simulink model "vertical_smm_3d_with_xz_lqr_with_torque_cmds"  (R2015a)
settings: Solver=FixedStepDiscrete  SolverMode=SingleTasking  StartTime=0.0  StopTime=inf  FixedStep=sample_time  RelTol=1e-3
values from neighbouring files (symbols this model uses):
  forward_dx_of_dxstar = [-1.33147741515 -1.28147741462 -1.23147741409 -1.18147741356 -1.13147741303 -1.0814774125 -1.03147741197 -0.981477411445 -0.931477410916 -0.881477410388 -0.831477409975 -0.781477409737 ... (28413 elements, 41x21x33)]    [ref_trajs.mat]
  forward_x_of_dxstar = [0.245075236011 0.237749717983 0.230424199955 0.223098681927 0.215773163898 0.20844764587 0.201122127842 0.193796609813 0.186471091785 0.179145573757 0.171820055745 0.164494537786 ... (28413 elements, 41x21x33)]    [ref_trajs.mat]
  target_dx_range = [-1 -0.95 -0.9 -0.85 -0.8 -0.75 -0.7 -0.65 -0.6 -0.55 -0.5 -0.45 ... (41 elements, 1x41)]    [ref_trajs.mat]
undefined symbols (not defined in the file or in its folder): A_kalman_fourbar_gear, A_kalman_transverse, A_kalman_vertical, A_lpf_accelerometer, A_lpf_dtau, A_lpf_fourbar_angles, A_lpf_imu, A_lpf_lateral_angle, A_lpf_leg_spring, B1_lpf_accelerometer, B1_lpf_dtau, B1_lpf_fourbar_angles, B1_lpf_imu, B1_lpf_lateral_angle, B1_lpf_leg_spring, B2_lpf_accelerometer, B2_lpf_dtau, B2_lpf_fourbar_angles, B2_lpf_imu, B2_lpf_lateral_angle, B2_lpf_leg_spring, B_dx_versus_x0, B_kalman_fourbar_gear, B_kalman_transverse, B_kalman_vertical, backwards_K_sag_of_t, backwards_P_sag_of_t, C_kalman_fourbar_gear, C_kalman_transverse, C_kalman_vertical, com_leg_motor, com_torso, contact_threshold, control_start_time, d_ankle_to_foot, d_vertical_com, desired_com_forward_velocity, desired_com_lateral_velocity, desired_initial_leg_roll_left, desired_initial_leg_roll_right, desired_stance_beta2, desired_standing_torso_pitch, desired_standing_torso_roll, desired_standing_z, desired_torso_pitch, desired_torso_roll, Discrete, enable_bouncing, enable_hopping, fcut_contact, g, HIP_MTR_MAX_CONT_TORQUE, HIP_MTR_MAX_TORQUE, i_leg_motor, i_robot, i_torso, initial_dx_estimate, initial_dy_estimate, initial_dz_estimate, initial_leg_selection ... (+77)
libraries: simulink x18, ctrlSharedLib x7
(part 3 of 5)

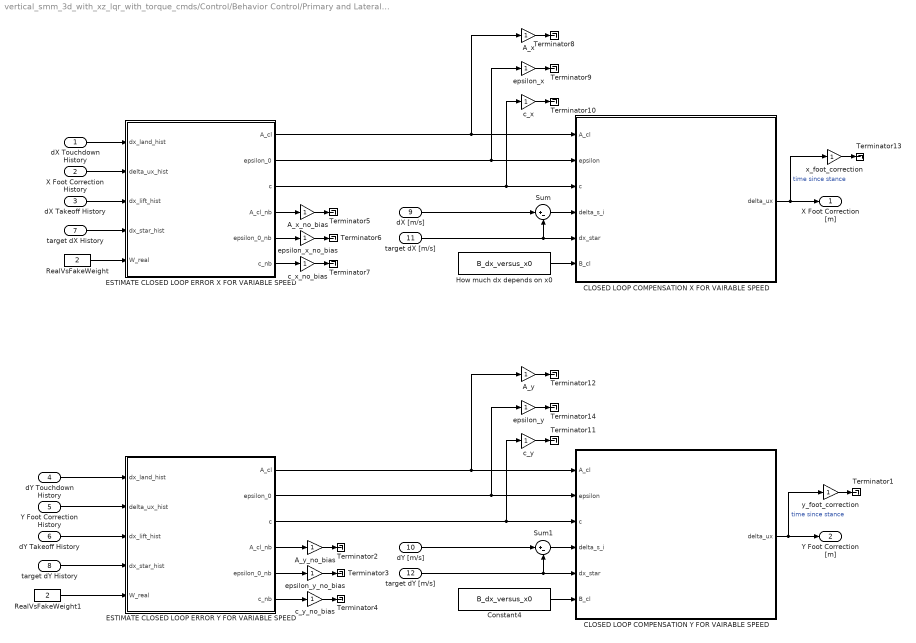
== system vertical_smm_3d_with_xz_lqr_with_torque_cmds/Control/Behavior Control/Primary and Lateral Behavior/Closed Loop Compensation ==
  dX Touchdown History : Inport
  X Foot Correction History : Inport  Port=2
  dX Takeoff History : Inport  Port=3
  dY Touchdown History : Inport  Port=4
  Y Foot Correction History : Inport  Port=5
  dY Takeoff History : Inport  Port=6
  target dX History : Inport  Port=7
  target dY History : Inport  Port=8
  dX [m/s] : Inport  Port=9
  dY [m/s] : Inport  Port=10
  target dX [m/s] : Inport  Port=11
  "target dY [m/s] " : Inport  Port=12
  A_x : Gain
  A_x_no_bias : Gain
  A_y : Gain
  A_y_no_bias : Gain
  CLOSED LOOP COMPENSATION X FOR VAIRABLE SPEED : MATLAB Function  TreatAsAtomicUnit=on
  CLOSED LOOP COMPENSATION Y FOR VAIRABLE SPEED : MATLAB Function  TreatAsAtomicUnit=on
  Constant4 : Constant  Value=B_dx_versus_x0
  ESTIMATE CLOSED LOOP ERROR X FOR VARIABLE SPEED : MATLAB Function  TreatAsAtomicUnit=on
  ESTIMATE CLOSED LOOP ERROR Y FOR VARIABLE SPEED : MATLAB Function  TreatAsAtomicUnit=on
  How much dx depends on x0 : Constant  Value=B_dx_versus_x0
  RealVsFakeWeight : Constant  Value=2
  RealVsFakeWeight1 : Constant  Value=2
  Sum : Sum  Inputs=|+-
  Sum1 : Sum  Inputs=|+-
  Terminator{1..14} (14 alike) : Terminator
  c_x : Gain
  c_x_no_bias : Gain
  c_y : Gain
  c_y_no_bias : Gain
  epsilon_x : Gain
  epsilon_x_no_bias : Gain
  epsilon_y : Gain
  epsilon_y_no_bias : Gain
  x_foot_correction : Gain
  y_foot_correction : Gain
  X Foot Correction [m] : Outport
  Y Foot Correction [m] : Outport  Port=2
  wires:
  RealVsFakeWeight1/1 -> ESTIMATE CLOSED LOOP ERROR Y FOR VARIABLE SPEED/5(W_real)
  Constant4/1 -> CLOSED LOOP COMPENSATION Y FOR VAIRABLE SPEED/6(B_cl)
  "target dY [m/s] "/1 -> Sum1/2, CLOSED LOOP COMPENSATION Y FOR VAIRABLE SPEED/5(dx_star)
  target dY History/1 -> ESTIMATE CLOSED LOOP ERROR Y FOR VARIABLE SPEED/4(dx_star_hist)
  Y Foot Correction History/1 -> ESTIMATE CLOSED LOOP ERROR Y FOR VARIABLE SPEED/2(delta_ux_hist)
  dY Takeoff History/1 -> ESTIMATE CLOSED LOOP ERROR Y FOR VARIABLE SPEED/3(dx_lift_hist)
  dY [m/s]/1 -> Sum1/1
  RealVsFakeWeight/1 -> ESTIMATE CLOSED LOOP ERROR X FOR VARIABLE SPEED/5(W_real)
  How much dx depends on x0/1 -> CLOSED LOOP COMPENSATION X FOR VAIRABLE SPEED/6(B_cl)
  Sum/1 -> CLOSED LOOP COMPENSATION X FOR VAIRABLE SPEED/4(delta_s_i)
  target dX [m/s]/1 -> Sum/2, CLOSED LOOP COMPENSATION X FOR VAIRABLE SPEED/5(dx_star)
  target dX History/1 -> ESTIMATE CLOSED LOOP ERROR X FOR VARIABLE SPEED/4(dx_star_hist)
  X Foot Correction History/1 -> ESTIMATE CLOSED LOOP ERROR X FOR VARIABLE SPEED/2(delta_ux_hist)
  dX Takeoff History/1 -> ESTIMATE CLOSED LOOP ERROR X FOR VARIABLE SPEED/3(dx_lift_hist)
  dX Touchdown History/1 -> ESTIMATE CLOSED LOOP ERROR X FOR VARIABLE SPEED/1(dx_land_hist)
  dX [m/s]/1 -> Sum/1
  dY Touchdown History/1 -> ESTIMATE CLOSED LOOP ERROR Y FOR VARIABLE SPEED/1(dx_land_hist)
  Sum1/1 -> CLOSED LOOP COMPENSATION Y FOR VAIRABLE SPEED/4(delta_s_i)
  CLOSED LOOP COMPENSATION X FOR VAIRABLE SPEED/1(delta_ux) -> x_foot_correction/1, X Foot Correction [m]/1  "time since stance"
  x_foot_correction/1 -> Terminator13/1
  CLOSED LOOP COMPENSATION Y FOR VAIRABLE SPEED/1(delta_ux) -> y_foot_correction/1, Y Foot Correction [m]/1  "time since stance"
  y_foot_correction/1 -> Terminator1/1
  ESTIMATE CLOSED LOOP ERROR X FOR VARIABLE SPEED/6(c_nb) -> c_x_no_bias/1
  ESTIMATE CLOSED LOOP ERROR X FOR VARIABLE SPEED/5(epsilon_0_nb) -> epsilon_x_no_bias/1
  ESTIMATE CLOSED LOOP ERROR X FOR VARIABLE SPEED/4(A_cl_nb) -> A_x_no_bias/1
  A_x_no_bias/1 -> Terminator5/1
  epsilon_x_no_bias/1 -> Terminator6/1
  c_x_no_bias/1 -> Terminator7/1
  A_y_no_bias/1 -> Terminator2/1
  epsilon_y_no_bias/1 -> Terminator3/1
  c_y_no_bias/1 -> Terminator4/1
  ESTIMATE CLOSED LOOP ERROR Y FOR VARIABLE SPEED/4(A_cl_nb) -> A_y_no_bias/1
  ESTIMATE CLOSED LOOP ERROR Y FOR VARIABLE SPEED/5(epsilon_0_nb) -> epsilon_y_no_bias/1
  ESTIMATE CLOSED LOOP ERROR Y FOR VARIABLE SPEED/6(c_nb) -> c_y_no_bias/1
  ESTIMATE CLOSED LOOP ERROR X FOR VARIABLE SPEED/3(c) -> c_x/1, CLOSED LOOP COMPENSATION X FOR VAIRABLE SPEED/3(c)
  ESTIMATE CLOSED LOOP ERROR X FOR VARIABLE SPEED/2(epsilon_0) -> epsilon_x/1, CLOSED LOOP COMPENSATION X FOR VAIRABLE SPEED/2(epsilon)
  ESTIMATE CLOSED LOOP ERROR X FOR VARIABLE SPEED/1(A_cl) -> A_x/1, CLOSED LOOP COMPENSATION X FOR VAIRABLE SPEED/1(A_cl)
  A_x/1 -> Terminator8/1
  epsilon_x/1 -> Terminator9/1
  c_x/1 -> Terminator10/1
  ESTIMATE CLOSED LOOP ERROR Y FOR VARIABLE SPEED/3(c) -> c_y/1, CLOSED LOOP COMPENSATION Y FOR VAIRABLE SPEED/3(c)
  ESTIMATE CLOSED LOOP ERROR Y FOR VARIABLE SPEED/2(epsilon_0) -> epsilon_y/1, CLOSED LOOP COMPENSATION Y FOR VAIRABLE SPEED/2(epsilon)
  ESTIMATE CLOSED LOOP ERROR Y FOR VARIABLE SPEED/1(A_cl) -> A_y/1, CLOSED LOOP COMPENSATION Y FOR VAIRABLE SPEED/1(A_cl)
  A_y/1 -> Terminator12/1
  epsilon_y/1 -> Terminator14/1
  c_y/1 -> Terminator11/1

== system vertical_smm_3d_with_xz_lqr_with_torque_cmds/Control/Behavior Control/Primary and Lateral Behavior/Enabled on Takeoff ==
  In : Inport
  Enable : EnablePort
  Out : Outport
  wires:
  In/1 -> Out/1

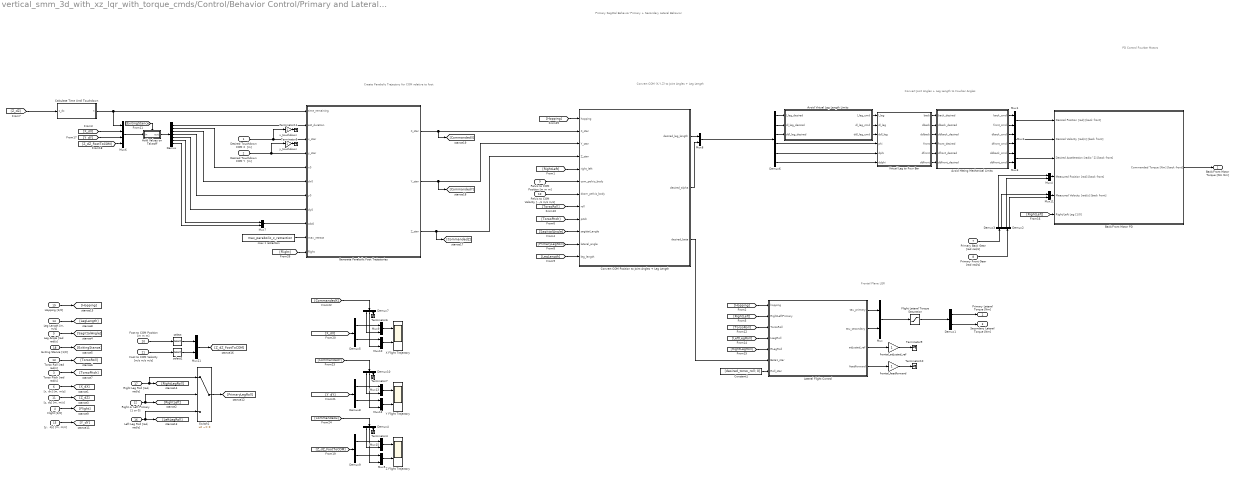
== system vertical_smm_3d_with_xz_lqr_with_torque_cmds/Control/Behavior Control/Primary and Lateral Behavior/Flight ==
  note: Primary Sagittal Behavior
      | Primary + Secondary Lateral Behavior
  note: Create Parabolic
      | Trajectory for COM relative to foot
  note: Convert COM (X,Y,Z) to
      | Joint Angles + Leg Length
  note: Convert Joint Angles + Leg Length
      | to Fourbar Angles
  note: PD Control Fourbar Motors
  note: Frontal Plane LQR
  Desired Touchdown COM X  [m] : Inport
  Desired Touchdown COM Y  [m] : Inport  Port=2
  Torso Pitch [rad rad/s] : Inport  Port=3
  Flight [1/0] : Inport  Port=4
  Leg Angle [rad rad/s] : Inport  Port=5
  "[x, dx] [m, m/s]" : Inport  Port=6
  Primary Back Gear [rad rad/s] : Inport  Port=7
  Primary Front Gear [rad rad/s] : Inport  Port=8
  Pelvis to COM Position [m m m] : Inport  Port=9
  Pelvis to COM Velocity [m/s m/s m/s] : Inport  Port=10
  "[z, dz] [m, m/s]" : Inport  Port=11
  Right or Left Primary [1 or 0] : Inport  Port=12
  Torso Roll [rad rad/s] : Inport  Port=13
  "Leg Length [m, m/s]" : Inport  Port=14
  "[y,  dy] [m, m/s]" : Inport  Port=15
  "Left Leg Roll [rad, rad/s]" : Inport  Port=16
  "Right Leg Roll [rad, rad/s]" : Inport  Port=17
  Exiting Stance [1/0] : Inport  Port=18
  Hopping [1/0] : Inport  Port=19
  Foot to COM Position [m m m] : Inport  Port=20
  Foot to COM Velocity [m/s m/s m/s] : Inport  Port=21
  Avoid Hitting Mechanical Limits : MATLAB Function  TreatAsAtomicUnit=on
  Avoid Virtual Leg Length Limits : MATLAB Function  TreatAsAtomicUnit=on
  Back/Front Motor PD : Subsystem
  Calculate Time Until Touchdown : MATLAB Function  TreatAsAtomicUnit=on
  Constant1 : Constant  Value=[desired_torso_roll; 0]
  "Convert COM Position to Joint Angles + Leg Length " : MATLAB Function  TreatAsAtomicUnit=on
  Demux : Demux  Outputs=7
  Demux{1..3,5,8..9} (6 alike) : Demux  Outputs=2
  Demux10 : Demux  Outputs=3
  Demux4 : Demux  Outputs=3
  Demux6 : Demux  Outputs=6
  Demux7 : Demux  Outputs=3
  Flight Lateral Torque Saturation : Saturate  UpperLimit=HIP_MTR_MAX_CONT_TORQUE  LowerLimit=-HIP_MTR_MAX_CONT_TORQUE
      settings: AttributesFormatString=Top: %<UpperLimit>\nBottom: %<LowerLimit>
  Generate Parabolic Foot Trajectories : MATLAB Function  TreatAsAtomicUnit=on
  Hold Values on Takeoff : Subsystem
  Lateral Flight Control : MATLAB Function  TreatAsAtomicUnit=on
  Mux{,1..5,7..13,15,21} (15 alike) : Mux  Inputs=2
  Mux6 : Mux
  Switch1 : Switch  Criteria=u2 ~= 0
  Terminator{4..7,9..11} (7 alike) : Terminator
  Virtual Leg to Four Bar : MATLAB Function  TreatAsAtomicUnit=on
  X Flight Trajectory : Scope  NumInputPorts=2
      settings: YMin=-1~-0.8  YMax=1~1.4  SaveName=ScopeData3  SampleInput=on
  Y Flight Trajectory : Scope  NumInputPorts=2
      settings: YMin=-1~-0.8  YMax=1~1.4  SaveName=ScopeData4  SampleInput=on
  Z Flight Trajectory : Scope  NumInputPorts=2
      settings: YMin=-1~-0.8  YMax=1~1.4  SaveName=ScopeData7  SampleInput=on
  frontal_adjusted_ref : Gain
  frontal_feedforward : Gain
  max z retraction : Constant  Value=max_parabolic_z_retraction
  select : Selector  InputPortWidth=3  Indices=[3]
  select1 : Selector  InputPortWidth=3  Indices=[3]
  x_touchdown : Gain
  y_touchdown : Gain
  Back/Front Motor Torque [Nm Nm] : Outport
  Primary Lateral Torque [Nm] : Outport  Port=2
  Secondary Lateral Torque [Nm] : Outport  Port=3
  wires:
  Virtual Leg to Four Bar/1(back) -> Avoid Hitting Mechanical Limits/1(back_desired)
  Virtual Leg to Four Bar/2(dback) -> Avoid Hitting Mechanical Limits/2(dback_desired)
  Virtual Leg to Four Bar/3(ddback) -> Avoid Hitting Mechanical Limits/3(ddback_desired)
  Virtual Leg to Four Bar/4(front) -> Avoid Hitting Mechanical Limits/4(front_desired)
  Virtual Leg to Four Bar/5(dfront) -> Avoid Hitting Mechanical Limits/5(dfront_desired)
  Virtual Leg to Four Bar/6(ddfront) -> Avoid Hitting Mechanical Limits/6(ddfront_desired)
  Mux11/1 -> Back/Front Motor PD/5(Measured Velocity [rad/s] [back front])
  Demux2/2 -> Mux11/2
  Mux4/1 -> Back/Front Motor PD/4(Measured Position [rad] [back front])
  Mux1/1 -> Back/Front Motor PD/1(Desired Position [rad] [back front])
  Demux3/2 -> Mux11/1
  Demux3/1 -> Mux4/1
  Avoid Hitting Mechanical Limits/2(front_cmd) -> Mux1/2
  Avoid Hitting Mechanical Limits/1(back_cmd) -> Mux1/1
  Demux2/1 -> Mux4/2
  Avoid Hitting Mechanical Limits/3(dback_cmd) -> Mux2/1
  Avoid Hitting Mechanical Limits/4(dfront_cmd) -> Mux2/2
  Avoid Hitting Mechanical Limits/5(ddback_cmd) -> Mux3/1
  Avoid Hitting Mechanical Limits/6(ddfront_cmd) -> Mux3/2
  Mux2/1 -> Back/Front Motor PD/2(Desired Velocity [rad/s] [back front])
  Mux3/1 -> Back/Front Motor PD/3(Desired Acceleration [rad/s^2] [back front])
  Back/Front Motor PD/1(Commanded Torque [Nm] [back front]) -> Back/Front Motor Torque [Nm Nm]/1
  Primary Back Gear [rad rad/s]/1 -> Demux3/1
  Primary Front Gear [rad rad/s]/1 -> Demux2/1
  [RightLeft] -> Back/Front Motor PD/6(Right/Left Leg [1/0])
  Demux/1 -> Generate Parabolic Foot Trajectories/2(est_duration)
  Mux7/1 -> Generate Parabolic Foot Trajectories/9(zdz0)
  max z retraction/1 -> Generate Parabolic Foot Trajectories/10(max_retract)
  Mux6/1 -> Hold Values on Takeoff/1(in)
  Hold Values on Takeoff/1(out) -> Demux/1
  [X_dX] -> Mux6/2
  Generate Parabolic Foot Trajectories/1(X_star) -> [CommandedX], "Convert COM Position to Joint Angles + Leg Length "/2(X_star)
  Generate Parabolic Foot Trajectories/2(Y_star) -> "Convert COM Position to Joint Angles + Leg Length "/3(Y_star), [CommandedY]
  [RightLeft] -> "Convert COM Position to Joint Angles + Leg Length "/5(right_left)
  "Convert COM Position to Joint Angles + Leg Length "/2(desired_alpha) -> Mux8/2
  "Convert COM Position to Joint Angles + Leg Length "/1(desired_leg_length) -> Mux8/1
  Demux6/6 -> Virtual Leg to Four Bar/6(ddphi)
  Demux6/5 -> Virtual Leg to Four Bar/5(dphi)
  Demux6/4 -> Virtual Leg to Four Bar/4(phi)
  Mux8/1 -> Demux6/1
  Leg Angle [rad rad/s]/1 -> [SagittalAngle]
  [SagittalAngle] -> "Convert COM Position to Joint Angles + Leg Length "/10(sagittal_angle)
  Torso Pitch [rad rad/s]/1 -> [TorsoPitch]
  [TorsoPitch] -> "Convert COM Position to Joint Angles + Leg Length "/9(pitch)
  [PrimaryLegRoll] -> "Convert COM Position to Joint Angles + Leg Length "/11(lateral_angle)
  [LegLength] -> "Convert COM Position to Joint Angles + Leg Length "/12(leg_length)
  [TorsoRoll] -> "Convert COM Position to Joint Angles + Leg Length "/8(roll)
  Pelvis to COM Position [m m m]/1 -> "Convert COM Position to Joint Angles + Leg Length "/6(com_pelvis_body)
  Pelvis to COM Velocity [m/s m/s m/s]/1 -> "Convert COM Position to Joint Angles + Leg Length "/7(dcom_pelvis_body)
  Flight [1/0]/1 -> [Flight]
  [ExitingStance] -> Hold Values on Takeoff/Trigger
  "[x, dx] [m, m/s]"/1 -> [X_dX]
  Torso Roll [rad rad/s]/1 -> [TorsoRoll]
  "Leg Length [m, m/s]"/1 -> [LegLength]
  "[z, dz] [m, m/s]"/1 -> [Z_dZ]
  Desired Touchdown COM X  [m]/1 -> Generate Parabolic Foot Trajectories/3(x_star), x_touchdown/1
  x_touchdown/1 -> Terminator11/1
  y_touchdown/1 -> Terminator5/1
  "[y,  dy] [m, m/s]"/1 -> [Y_dY]
  [Y_dY] -> Mux6/3
  [Z_dZ] -> Calculate Time Until Touchdown/1(z_dz)
  Calculate Time Until Touchdown/1(t) -> Mux6/1, Generate Parabolic Foot Trajectories/1(time_remaining)
  Avoid Virtual Leg Length Limits/1(l_leg_cmd) -> Virtual Leg to Four Bar/1(l_leg)
  Avoid Virtual Leg Length Limits/2(dl_leg_cmd) -> Virtual Leg to Four Bar/2(dl_leg)
  Avoid Virtual Leg Length Limits/3(ddl_leg_cmd) -> Virtual Leg to Four Bar/3(ddl_leg)
  Demux6/1 -> Avoid Virtual Leg Length Limits/1(l_leg_desired)
  Demux6/2 -> Avoid Virtual Leg Length Limits/2(dl_leg_desired)
  Demux6/3 -> Avoid Virtual Leg Length Limits/3(ddl_leg_desired)
  Desired Touchdown COM Y  [m]/1 -> y_touchdown/1, Generate Parabolic Foot Trajectories/4(y_star)
  [RightLeft] -> Lateral Flight Control/2(RightLeftPrimary)
  [TorsoRoll] -> Lateral Flight Control/3(TorsoRoll)
  Constant1/1 -> Lateral Flight Control/7(Roll_star)
  Lateral Flight Control/3(adjusted_ref) -> frontal_adjusted_ref/1
  Lateral Flight Control/4(feedforward) -> frontal_feedforward/1
  Lateral Flight Control/2(tau_secondary) -> Mux/2
  Lateral Flight Control/1(tau_primary) -> Mux/1
  "Left Leg Roll [rad, rad/s]"/1 -> Switch1/3, [LeftLegRoll]
  [LeftLegRoll] -> Lateral Flight Control/4(LLegRoll)
  [RightLegRoll] -> Lateral Flight Control/5(RLegRoll)
  "Right Leg Roll [rad, rad/s]"/1 -> Switch1/1, [RightLegRoll]
  Right or Left Primary [1 or 0]/1 -> Switch1/2, [RightLeft]
  Switch1/1 -> [PrimaryLegRoll]
  Exiting Stance [1/0]/1 -> [ExitingStance]
  Demux1/1 -> Primary Lateral Torque [Nm]/1
  Demux1/2 -> Secondary Lateral Torque [Nm]/1
  "Convert COM Position to Joint Angles + Leg Length "/3(desired_beta) -> Lateral Flight Control/6(Beta1_star)
  Flight Lateral Torque Saturation/1 -> Demux1/1
  frontal_feedforward/1 -> Terminator10/1
  frontal_adjusted_ref/1 -> Terminator9/1
  [Hopping] -> "Convert COM Position to Joint Angles + Leg Length "/1(hopping)
  Mux/1 -> Flight Lateral Torque Saturation/1
  [Hopping] -> Lateral Flight Control/1(hopping)
  Hopping [1/0]/1 -> [Hopping]
  [Flight] -> Generate Parabolic Foot Trajectories/11(flight)
  Demux/2 -> Generate Parabolic Foot Trajectories/5(x0)
  Demux/3 -> Generate Parabolic Foot Trajectories/6(dx0)
  Demux/4 -> Generate Parabolic Foot Trajectories/7(y0)
  Demux/5 -> Generate Parabolic Foot Trajectories/8(dy0)
  Demux/6 -> Mux7/1
  Demux/7 -> Mux7/2
  Foot to COM Position [m m m]/1 -> select/1
  Foot to COM Velocity [m/s m/s m/s]/1 -> select1/1
  select/1 -> Mux21/1
  select1/1 -> Mux21/2
  Mux21/1 -> [Z_dZ_FootToCOM]
  Mux15/1 -> Z Flight Trajectory/1
  Mux5/1 -> Z Flight Trajectory/2
  [Z_dZ_FootToCOM] -> Mux6/4
  [Z_dZ_FootToCOM] -> Demux9/1
  Demux9/1 -> Mux15/1
  Demux9/2 -> Mux5/1
  Demux4/1 -> Mux15/2
  Demux4/2 -> Mux5/2
  Demux4/3 -> Terminator4/1
  Mux9/1 -> X Flight Trajectory/1
  Mux10/1 -> X Flight Trajectory/2
  Demux5/1 -> Mux9/1
  Demux5/2 -> Mux10/1
  Demux7/1 -> Mux9/2
  Demux7/2 -> Mux10/2
  [X_dX] -> Demux5/1
  Demux7/3 -> Terminator6/1
  Mux13/1 -> Y Flight Trajectory/1
  Mux12/1 -> Y Flight Trajectory/2
  Demux8/1 -> Mux13/1
  Demux8/2 -> Mux12/1
  Demux10/1 -> Mux13/2
  Demux10/2 -> Mux12/2
  [Y_dY] -> Demux8/1
  Demux10/3 -> Terminator7/1
  [CommandedX] -> Demux7/1
  [CommandedY] -> Demux10/1
  [CommandedZ] -> Demux4/1
  Generate Parabolic Foot Trajectories/3(Z_star) -> "Convert COM Position to Joint Angles + Leg Length "/4(Z_star), [CommandedZ]

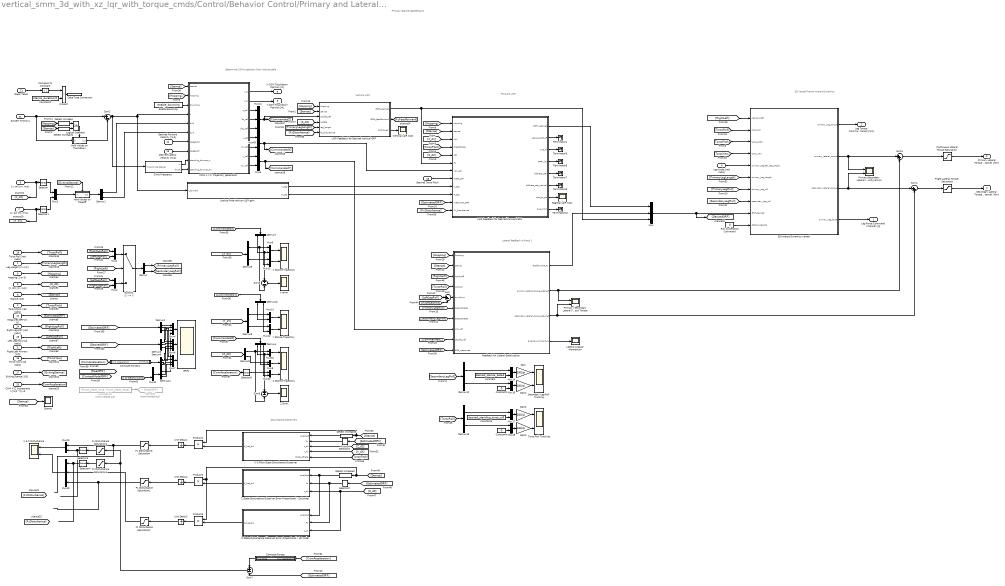
== system vertical_smm_3d_with_xz_lqr_with_torque_cmds/Control/Behavior Control/Primary and Lateral Behavior/Stance ==
  note: Lateral feedback without Y
  note: 3D Yawed Frame Inverse Dynamics
  note: Forward LQR
  note: Vertical LQR
  note: Determine COM trajectory
      | from lookup table
  note: Primary Stance Leg Behavior
  note: Disturbance Observers
  Leg Length [m m/s] : Inport
  Torso Pitch [rad rad/s] : Inport  Port=2
  Stance [1/0] : Inport  Port=3
  Leg Angle [rad rad/s] : Inport  Port=4
  Right/Left Primary [1/0] : Inport  Port=5
  "[x, dx] [m, m/s]" : Inport  Port=6
  "[y, dy] [m, m/s]" : Inport  Port=7
  "[z, dz] [m, m/s]" : Inport  Port=8
  Hopping [1 or 0] : Inport  Port=9
  Measured GRF [N N] : Inport  Port=10
  Steps Taken : Inport  Port=11
  Desired Forward Velocity [m/s] : Inport  Port=12
  Desired Lateral Velocity [m/s] : Inport  Port=13
  Right Leg Roll [rad rad/s] : Inport  Port=14
  Left Leg Roll [rad rad/s] : Inport  Port=15
  Torso Yaw [rad rad/s] : Inport  Port=16
  Exiting Stance [1/0] : Inport  Port=17
  Desired Torso Pitch : Inport  Port=18
  Torso Roll [rad rad/s] : Inport  Port=19
  COM XYZ Acceleration [m/s^2] x3 : Inport  Port=20
  System Time [s] : Inport  Port=21
  3D Inverse Dynamics yawed : MATLAB Function  TreatAsAtomicUnit=on
  COM X,Y,Z  trajectory generation : MATLAB Function  TreatAsAtomicUnit=on
  Chirp Frequency : Subsystem
  Compare To Constant : simulink/Logic and Bit Operations/Compare To Constant  relop=<  const=1  OutDataTypeStr=uint8
  Compute Forces : Subsystem
  Compute Forces1 : Subsystem
  Constant : Constant  Value=desired_stance_beta2
  Constant1 : Constant  Value=0
  Constant2 : Constant  Value=stance_duration/2
  Constant3 : Constant  Value=desired_standing_torso_roll
  Constant4 : Constant  Value=0
  Continuous Lateral Torque Saturation : Saturate  UpperLimit=max_primary_lateral_stance_torque  LowerLimit=-max_primary_lateral_stance_torque
      settings: AttributesFormatString=Top: %<UpperLimit>\nBottom: %<LowerLimit>
  Data Type Conversion : DataTypeConversion  OutDataTypeStr=double
  Demux{,1,5,7..10,12..13} (9 alike) : Demux  Outputs=2
  Demux{2..4,6,11} (5 alike) : Demux  Outputs=3
  Detect Increase{,1..3} (4 alike) : simulink/Logic and Bit Operations/Detect Increase  vinit=0.0  InputProcessing=Inherited  OutDataTypeStr=boolean
  Enable Bouncing : Constant  Value=enable_bouncing  SampleTime=sample_time
  Feedback for Lateral Stabilization : MATLAB Function  TreatAsAtomicUnit=on
  Flight Lateral Torque Saturation : Saturate  UpperLimit=HIP_MTR_MAX_CONT_TORQUE  LowerLimit=-HIP_MTR_MAX_CONT_TORQUE
      settings: AttributesFormatString=Top: %<UpperLimit>\nBottom: %<LowerLimit>
  Fx Disturbance Saturation : Saturate  UpperLimit=100  LowerLimit=-100
      settings: AttributesFormatString=Top: %<UpperLimit>\nBottom: %<LowerLimit>
  Fx Disturbance Saturation1 : Saturate  UpperLimit=100  LowerLimit=-100
      settings: AttributesFormatString=Top: %<UpperLimit>\nBottom: %<LowerLimit>
  Fz Disturbance Saturation1 : Saturate  UpperLimit=100  LowerLimit=-100
      settings: AttributesFormatString=Top: %<UpperLimit>\nBottom: %<LowerLimit>
  Fz Disturbance Saturation2 : Saturate  UpperLimit=100  LowerLimit=-100
      settings: AttributesFormatString=Top: %<UpperLimit>\nBottom: %<LowerLimit>
  Fz Disturbance Saturation4 : Saturate  UpperLimit=100  LowerLimit=-100
      settings: AttributesFormatString=Top: %<UpperLimit>\nBottom: %<LowerLimit>
  GRFs : Scope  NumInputPorts=3
      settings: TimeRange=37.999  YMin=-1250~-2000~-1250  YMax=1500~3750~1750  SampleInput=on
  Gain{,1..3} (4 alike) : Gain  Gain=180/pi
  Hold Values on Takeoff : Subsystem
  Hold Values on Touchdown : Subsystem
  LQR Feedback for Desired Forward GRF : MATLAB Function  TreatAsAtomicUnit=on
  LQR Feedback for Desired Vertical GRF : MATLAB Function  TreatAsAtomicUnit=on
  Lateral Angular Momentum : Scope
      settings: YMin=-3.5  YMax=4  SaveName=ScopeData20  SampleInput=on
  Logical Operator : Logic  Operator=OR  AllPortsSameDT=off  OutDataTypeStr=boolean
  Lookup finite horizon LQR gain : MATLAB Function  TreatAsAtomicUnit=on
  Mux{,11,19,21} (4 alike) : Mux  Inputs=3
  Mux{1..3,5,8..10,12..18,20,22,49} (17 alike) : Mux  Inputs=2
  Mux4 : Mux
  Mux6 : Mux
  Mux7 : Mux
  Primary / Secondary Lateral Feedback Torque : Scope  NumInputPorts=2
      settings: YMin=-3.5~-5  YMax=4~5  SaveName=ScopeData9  SampleInput=on
  Primary/Secondary Lateral Inverse Dynamics : Scope  NumInputPorts=2
      settings: YMin=40~-5  YMax=150~5  SaveName=ScopeData34  SampleInput=on
  Product{,1..3} (4 alike) : Product
  Roll Accleration Command : Constant  Value=0
  Sagittal LQR Cost : Scope
      settings: YMin=22.5  YMax=62.5  SaveName=ScopeData10  SampleInput=on
  Secondary Leg Roll Tracking : Scope  NumInputPorts=2
      settings: YMin=-3.5~-5  YMax=4~5  SaveName=ScopeData12  SampleInput=on
  Selector : Selector  InputPortWidth=2  Indices=[2]
  Selector1 : Selector  InputPortWidth=2  Indices=[2]
  Selector2 : Selector  InputPortWidth=3  Indices=[3]
  Selector3 : Selector  InputPortWidth=3  Indices=[1]
  Selector4 : Selector  InputPortWidth=3  Indices=[3]
  Selector5 : Selector  InputPortWidth=3  Indices=[1]
  Selector6 : Selector  InputPortWidth=3  Indices=[3]
  Stance : Scope
      settings: YMin=-0.05  YMax=0.11  SaveName=stance_time_history  SampleInput=on
  Sum : Sum  Inputs=|+-
  Sum2 : Sum  Inputs=|+-
  Sum3 : Sum  Inputs=|++
  Sum4 : Sum  Inputs=|++
  Sum5 : Sum  Inputs=+-
  Sum6 : Sum  Inputs=+-
  Sum7 : Sum  Inputs=+-
  Switch1 : Switch  Criteria=u2 ~= 0
  Terminator{4..8,10} (6 alike) : Terminator
  Torso Roll Tracking : Scope  NumInputPorts=2
      settings: YMin=-3.5~-5  YMax=4~5  SaveName=ScopeData15  SampleInput=on
  Unit Delay1 : UnitDelay  SampleTime=sample_time
  Unit Delay2 : UnitDelay  SampleTime=sample_time
  Unit Delay3 : UnitDelay  SampleTime=sample_time
  Vertical LQR Cost : Scope
      settings: YMin=11  YMax=16  SaveName=ScopeData18  SampleInput=on
  X & Pitch State Disturbance Observer : MATLAB Function  TreatAsAtomicUnit=on
  X & Z Disturbance : Scope  NumInputPorts=2
      settings: YMin=-125~-800  YMax=175~700  SaveName=ScopeData16  SampleInput=on
  X Stance Trajectory : Scope  NumInputPorts=2
      settings: YMin=0~-0.02  YMax=0.005~0.03  SaveName=ScopeData8  SampleInput=on
  X error : Scope
      settings: YMin=-0.05  YMax=0.11  SaveName=ScopeData24  SampleInput=on
  Y Stance Trajectory : Scope  NumInputPorts=2
      settings: YMin=0.005~-0.5  YMax=0.1~0.3  SaveName=ScopeData5  SampleInput=on
  Z Error : Scope
      settings: YMin=-0.007  YMax=0.0005  SaveName=ScopeData23  SampleInput=on
  Z Stance Trajectory : Scope  NumInputPorts=3
      settings: YMin=0.85~-0.4~-3  YMax=0.98~0.6~11  SaveName=z_stance_trajectory  SampleInput=on
  Z State Disturbance Observer Error-Proportional - 1st order : MATLAB Function  TreatAsAtomicUnit=on
  Z State Disturbance Observer Error-Proportional - 2nd order : MATLAB Function  TreatAsAtomicUnit=on
  recorded q1 : FromWorkspace  Commented=on  VariableName=[force_plate_time, force_plate_data]  OutDataTypeStr=double  OutputAfterFinalValue=Holding final value
  stance20 : Goto  Commented=on  GotoTag=RealGRF
  Leg Force Command (stance) [N] : Outport
  Leg Torque Command (stance) [Nm] : Outport  Port=2
  Primary Lateral Torque Command (stance) [Nm] : Outport  Port=3
  Secondary Lateral Torque Command (stance) [Nm] : Outport  Port=4
  X COM Touchdown Position [m] : Outport  Port=5
  Y COM Touchdown Position [m] : Outport  Port=6
  wires:
  Fz Disturbance Saturation4/1 -> Selector4/1
  Fz Disturbance Saturation1/1 -> Mux19/3
  Fx Disturbance Saturation1/1 -> Selector5/1
  Chirp Frequency/2(dw/dt) -> COM X,Y,Z  trajectory generation/10(standing_bounce_dw)
  [Stance] -> Stance/1
  Chirp Frequency/1(w) -> COM X,Y,Z  trajectory generation/9(standing_bounce_w)
  Selector2/1 -> Z State Disturbance Observer Error-Proportional - 1st order/2(Fz), Z State Disturbance Observer Error-Proportional - 2nd order/2(Fz)
  Sum7/1 -> Fx Disturbance Saturation1/1, Fz Disturbance Saturation4/1
  Unit Delay3/1 -> Fz Disturbance Saturation2/1
  Selector5/1 -> Mux20/2
  Mux20/1 -> X & Z Disturbance/1
  [ComAcceleration] -> Compute Forces/1(XYZ Acceleration)
  Compute Forces/1(XYZ Force) -> Sum7/1
  [FxDisturbance] -> LQR Feedback for Desired Forward GRF/12(Fx_disturbance)
  Sum6/1 -> X error/1
  Demux7/1 -> Mux9/2, Sum6/1
  Demux5/1 -> Mux9/1, Sum6/2
  Unit Delay2/1 -> Fz Disturbance Saturation1/1
  Unit Delay1/1 -> Fx Disturbance Saturation/1
  Selector3/1 -> X & Pitch State Disturbance Observer/2(Fx)
  Fx Disturbance Saturation/1 -> Mux20/1
  Enable Bouncing/1 -> COM X,Y,Z  trajectory generation/3(bouncing)
  [RightLeft] -> Feedback for Lateral Stabilization/3(right_left)
  Constant4/1 -> Mux18/2
  Mux18/1 -> Gain3/1
  Demux13/2 -> Mux18/1
  Constant3/1 -> Mux17/2
  Demux13/1 -> Mux17/1
  Mux17/1 -> Gain2/1
  Gain3/1 -> Torso Roll Tracking/2
  Gain2/1 -> Torso Roll Tracking/1
  [TorsoRoll] -> Demux13/1
  Constant1/1 -> Mux16/2
  Demux12/2 -> Mux16/1
  Mux16/1 -> Gain1/1
  Gain1/1 -> Secondary Leg Roll Tracking/2
  Gain/1 -> Secondary Leg Roll Tracking/1
  Constant/1 -> Mux14/2
  Demux12/1 -> Mux14/1
  Mux14/1 -> Gain/1
  [SecondaryLegRoll] -> Demux12/1
  Feedback for Lateral Stabilization/3(secondary_lateral_torque_desired) -> Sum4/2, Primary / Secondary Lateral Feedback Torque/2
  Sum4/1 -> Flight Lateral Torque Saturation/1
  3D Inverse Dynamics yawed/2(primary_lateral_torque) -> Sum3/1, Primary/Secondary Lateral Inverse Dynamics/1
  3D Inverse Dynamics yawed/3(secondary_lateral_torque) -> Sum4/1, Primary/Secondary Lateral Inverse Dynamics/2
  Sum/1 -> Feedback for Lateral Stabilization/5(symdsym)
  [SecondaryLegRoll] -> Feedback for Lateral Stabilization/7(beta2dbeta2)
  [PrimaryLegRoll] -> Feedback for Lateral Stabilization/6(beta1dbeta1)
  [RightLegRoll] -> Sum/2
  [LeftLegRoll] -> Sum/1
  Feedback for Lateral Stabilization/2(primary_lateral_torque_desired) -> Sum3/2, Primary / Secondary Lateral Feedback Torque/1
  Sum3/1 -> Continuous Lateral Torque Saturation/1
  Roll Accleration Command/1 -> 3D Inverse Dynamics yawed/10(ddRoll_desired)
  Feedback for Lateral Stabilization/1(feedforward_Fy) -> Mux/2
  Continuous Lateral Torque Saturation/1 -> Primary Lateral Torque Command (stance) [Nm]/1
  Demux11/3 -> Mux7/4
  Demux11/2 -> Mux6/4
  Demux11/1 -> Mux4/4
  Mux/1 -> [DesiredGRF], 3D Inverse Dynamics yawed/9(GRF_desired)
  LQR Feedback for Desired Forward GRF/1(GRFx_desired) -> Mux/1
  Left Leg Roll [rad rad/s]/1 -> [LeftLegRoll]
  Right/Left Primary [1/0]/1 -> [RightLeft]
  [CommandedY] -> Demux10/1
  [CommandedX] -> Demux7/1
  [Y_dY] -> Demux8/1
  Demux10/2 -> Mux12/2
  Demux10/1 -> Mux13/2
  Demux8/2 -> Mux12/1
  Demux8/1 -> Mux13/1
  Mux12/1 -> Y Stance Trajectory/2
  Mux13/1 -> Y Stance Trajectory/1
  [X_dX] -> Demux5/1
  Demux7/2 -> Mux10/2
  Demux5/2 -> Mux10/1
  Mux10/1 -> X Stance Trajectory/2
  Mux9/1 -> X Stance Trajectory/1
  Demux3/3 -> Mux7/2
  Demux3/2 -> Mux6/2
  Demux3/1 -> Mux4/2
  Demux2/3 -> Mux7/1
  Demux2/2 -> Mux6/1
  Mux7/1 -> GRFs/3
  Mux6/1 -> GRFs/2
  Demux2/1 -> Mux4/1
  Mux4/1 -> GRFs/1
  [DesiredGRF] -> Demux3/1
  [EstimatedGRF] -> Demux2/1
  Torso Roll [rad rad/s]/1 -> [TorsoRoll]
  [PrimaryLegLength] -> LQR Feedback for Desired Vertical GRF/5(leg_length)
  Leg Length [m m/s]/1 -> [PrimaryLegLength]
  System Time [s]/1 -> Sum2/1, Hold Values on Touchdown/1(in)
  [EstimatedGRF] -> Feedback for Lateral Stabilization/10(GRF_measured)
  [Hopping] -> Feedback for Lateral Stabilization/1(hopping)
  3D Inverse Dynamics yawed/4(primary_leg_force) -> Leg Force Command (stance) [N]/1
  [ExitingStance] -> Hold Values on Takeoff/Trigger
  Exiting Stance [1/0]/1 -> [ExitingStance]
  Torso Yaw [rad rad/s]/1 -> [TorsoYaw]
  Desired Lateral Velocity [m/s]/1 -> COM X,Y,Z  trajectory generation/8(target_DY)
  Selector1/1 -> Mux3/2
  Hold Values on Takeoff/1(out) -> Demux1/1
  Mux3/1 -> Hold Values on Takeoff/1(in)
  "[y, dy] [m, m/s]"/1 -> Selector1/1, [Y_dY]
  [RightLeft] -> Switch1/2
  [RightLegRoll] -> Mux2/2
  [LeftLegRoll] -> Mux2/1
  [LeftLegRoll] -> Mux1/2
  [RightLegRoll] -> Mux1/1
  Right Leg Roll [rad rad/s]/1 -> [RightLegRoll]
  Mux2/1 -> Switch1/3
  Mux1/1 -> Switch1/1
  Demux/1 -> [PrimaryLegRoll]
  Demux/2 -> [SecondaryLegRoll]
  Switch1/1 -> Demux/1
  [PrimaryLegRoll] -> 3D Inverse Dynamics yawed/7(primary_leg_roll)
  [SecondaryLegRoll] -> 3D Inverse Dynamics yawed/8(secondary_leg_roll)
  Leg Angle [rad rad/s]/1 -> 3D Inverse Dynamics yawed/5(primary_sagittal_leg_angle)
  [PrimaryLegLength] -> 3D Inverse Dynamics yawed/6(primary_leg_length)
  [TorsoYaw] -> 3D Inverse Dynamics yawed/4(torso_yaw)
  [TorsoRoll] -> 3D Inverse Dynamics yawed/2(torso_roll)
  [TorsoPitch] -> 3D Inverse Dynamics yawed/3(torso_pitch)
  Mux5/1 -> [CommandedY], Feedback for Lateral Stabilization/8(ydy_ref)
  COM X,Y,Z  trajectory generation/2(y_0) -> Y COM Touchdown Position [m]/1
  [CommandedZ] -> Feedback for Lateral Stabilization/9(zdzddz_ref)
  [TorsoRoll] -> Feedback for Lateral Stabilization/4(rolldroll)
  [Stance] -> Feedback for Lateral Stabilization/2(stance)
  [Hopping] -> LQR Feedback for Desired Vertical GRF/1(hopping)
  Selector/1 -> Mux3/1
  Demux1/1 -> COM X,Y,Z  trajectory generation/5(dx0)
  [Stance] -> Detect Increase1/1
  [Hopping] -> Detect Increase/1
  Compare To Constant/1 -> Product/1
  Detect Increase1/1 -> Logical Operator/2
  Detect Increase/1 -> Logical Operator/1
  Constant2/1 -> Product/2
  Product/1 -> Data Type Conversion/1
  Steps Taken/1 -> Compare To Constant/1
  [EstimatedGRF] -> LQR Feedback for Desired Forward GRF/11(measured_GRF)
  Measured GRF [N N]/1 -> [EstimatedGRF]
  [Hopping] -> LQR Feedback for Desired Forward GRF/1(hopping)
  [Hopping] -> COM X,Y,Z  trajectory generation/2(hopping)
  Hopping [1 or 0]/1 -> [Hopping]
  [RightLeft] -> 3D Inverse Dynamics yawed/1(right_or_left)
  Torso Pitch [rad rad/s]/1 -> [TorsoPitch]
  LQR Feedback for Desired Forward GRF/8(ang_mom) -> Terminator10/1
  LQR Feedback for Desired Forward GRF/7(cost_to_go) -> Sagittal LQR Cost/1
  LQR Feedback for Desired Forward GRF/6(ddtheta_star_neutral) -> Terminator8/1
  LQR Feedback for Desired Forward GRF/5(ddtheta_star) -> Terminator7/1
  LQR Feedback for Desired Forward GRF/3(true_ff) -> Terminator5/1
  LQR Feedback for Desired Forward GRF/2(netural_pitch_ff) -> Terminator4/1
  LQR Feedback for Desired Vertical GRF/3(cost_to_go) -> Vertical LQR Cost/1
  Demux1/2 -> COM X,Y,Z  trajectory generation/6(dy0)
  "[x, dx] [m, m/s]"/1 -> Selector/1, [X_dX]
  Logical Operator/1 -> Hold Values on Touchdown/Trigger
  [Stance] -> LQR Feedback for Desired Vertical GRF/2(stance)
  Stance [1/0]/1 -> [Stance]
  Hold Values on Touchdown/1(out) -> Sum2/2
  LQR Feedback for Desired Vertical GRF/1(GRFz_desired) -> Mux/3, LQR Feedback for Desired Forward GRF/6(Fz)
  Sum2/1 -> COM X,Y,Z  trajectory generation/4(t), Lookup finite horizon LQR gain/1(t_forward), Chirp Frequency/1(Time Since Stance)
  Desired Forward Velocity [m/s]/1 -> COM X,Y,Z  trajectory generation/7(target_DX)
  [Z_dZ] -> LQR Feedback for Desired Forward GRF/5(zdz)
  Lookup finite horizon LQR gain/1(K_sag) -> LQR Feedback for Desired Forward GRF/9(K_sag)
  Desired Torso Pitch/1 -> LQR Feedback for Desired Forward GRF/8(theta_star)
  Mux49/1 -> LQR Feedback for Desired Forward GRF/7(xdx_ref), [CommandedX]
  [TorsoPitch] -> LQR Feedback for Desired Forward GRF/4(thetadtheta)
  [X_dX] -> LQR Feedback for Desired Forward GRF/3(xdx)
  Mux11/1 -> LQR Feedback for Desired Vertical GRF/3(zdzddz_ref), [CommandedZ]
  COM X,Y,Z  trajectory generation/5(ddz_ref) -> Mux11/3
  COM X,Y,Z  trajectory generation/4(dz_ref) -> Mux11/2
  COM X,Y,Z  trajectory generation/1(x_0) -> X COM Touchdown Position [m]/1
  COM X,Y,Z  trajectory generation/9(dy_ref) -> Mux5/2
  COM X,Y,Z  trajectory generation/8(y_ref) -> Mux5/1
  COM X,Y,Z  trajectory generation/7(dx_ref) -> Mux49/2
  COM X,Y,Z  trajectory generation/6(x_ref) -> Mux49/1
  [Stance] -> LQR Feedback for Desired Forward GRF/2(stance)
  COM X,Y,Z  trajectory generation/3(z_ref) -> Mux11/1
  [Z_dZ] -> LQR Feedback for Desired Vertical GRF/4(z_state)
  3D Inverse Dynamics yawed/1(primary_leg_torque) -> Leg Torque Command (stance) [Nm]/1
  Lookup finite horizon LQR gain/2(P_sag) -> LQR Feedback for Desired Forward GRF/10(P_sag)
  [Stance] -> COM X,Y,Z  trajectory generation/1(stance)
  LQR Feedback for Desired Forward GRF/4(GRFx_lqr) -> Terminator6/1
  Feedback for Lateral Stabilization/4(angular_momentum) -> Lateral Angular Momentum/1
  Demux6/1 -> Mux4/3
  Demux6/2 -> Mux6/3
  Demux6/3 -> Mux7/3
  Flight Lateral Torque Saturation/1 -> Secondary Lateral Torque Command (stance) [Nm]/1
  "[z, dz] [m, m/s]"/1 -> [Z_dZ]
  [Z_dZ] -> X & Pitch State Disturbance Observer/3(z_dz)
  [TorsoPitch] -> X & Pitch State Disturbance Observer/5(theta_dtheta)
  [X_dX] -> X & Pitch State Disturbance Observer/4(x_dx)
  [EstimatedGRF] -> Selector3/1
  Detect Increase3/1 -> X & Pitch State Disturbance Observer/1(enabled)
  Detect Increase2/1 -> Z State Disturbance Observer Error-Proportional - 1st order/1(enabled), Z State Disturbance Observer Error-Proportional - 2nd order/1(enabled)
  [EstimatedGRF] -> Selector2/1
  [Z_dZ] -> Z State Disturbance Observer Error-Proportional - 1st order/3(z_dz), Z State Disturbance Observer Error-Proportional - 2nd order/3(z_dz)
  Product1/1 -> Unit Delay1/1
  Product2/1 -> Unit Delay2/1
  X & Pitch State Disturbance Observer/1(d_hat_tp1) -> Product1/2
  [Stance] -> Product1/1, Detect Increase3/1
  Z State Disturbance Observer Error-Proportional - 2nd order/1(d_hat_tp1) -> Product2/2
  Product3/1 -> Unit Delay3/1
  Z State Disturbance Observer Error-Proportional - 1st order/1(d_hat_tp1) -> Product3/2
  [Stance] -> Product3/1, Product2/1, Detect Increase2/1
  Mux19/1 -> X & Z Disturbance/2
  Fz Disturbance Saturation2/1 -> Mux19/2
  [EstimatedGRF] -> Sum7/2
  Selector4/1 -> Mux19/1
  recorded q1/1 -> stance20/1
  COM XYZ Acceleration [m/s^2] x3/1 -> [ComAcceleration]
  [ComAcceleration] -> Compute Forces1/1(XYZ Acceleration)
  Compute Forces1/1(XYZ Force) -> Demux6/1
  [FzDisturbance] -> LQR Feedback for Desired Vertical GRF/6(Fz_disturbance)
  LQR Feedback for Desired Vertical GRF/2(GRFz_feedforward) -> [FzFeedforward]
  Mux21/1 -> Demux11/1
  [FzFeedforward] -> Mux21/3
  Mux15/1 -> Z Stance Trajectory/1
  Mux8/1 -> Z Stance Trajectory/2
  [Z_dZ] -> Demux9/1
  Demux9/1 -> Mux15/1, Sum5/2
  Demux9/2 -> Mux8/1
  Demux4/1 -> Mux15/2, Sum5/1
  Demux4/2 -> Mux8/2
  Demux4/3 -> Mux22/2
  [CommandedZ] -> Demux4/1
  Sum5/1 -> Z Error/1
  Mux22/1 -> Z Stance Trajectory/3
  [ComAcceleration] -> Selector6/1
  Selector6/1 -> Mux22/1

== system vertical_smm_3d_with_xz_lqr_with_torque_cmds/Control/Behavior Control/Secondary Leg Behavior/Back//Front Motor PD ==
  Desired Position [rad] [back front] : Inport
  Desired Velocity [rad/s] [back front] : Inport  Port=2
  Desired Acceleration [rad/s^2] [back front] : Inport  Port=3
  Measured Position [rad] [back front] : Inport  Port=4
  Measured Velocity [rad/s] [back front] : Inport  Port=5
  Right/Left Leg [1/0] : Inport  Port=6
  Divide : Product  Inputs=*/
  Friction Compensation : Subsystem
  Load Torque in Flight : Constant  Value=30
  Motor Efficiency : MATLAB Function  TreatAsAtomicUnit=on
  Product : Product
  RPM in Flight : Constant  Value=0
  Sum1 : Sum  Inputs=|++
  Sum2 : Sum  Inputs=|++
  Sum7 : Sum  Inputs=|+-
  Sum8 : Sum  Inputs=|+-
  Sum9 : Sum
  kd : Gain  Gain=kd_motor
  kp : Gain  Gain=kp_motor
  reflected inertia : Constant  Value=j_motor
  Commanded Torque [Nm] [back front] : Outport
  wires:
  kp/1 -> Sum9/1
  Sum7/1 -> kp/1
  Measured Position [rad] [back front]/1 -> Sum7/2
  Sum9/1 -> Sum1/1
  Sum8/1 -> kd/1
  Desired Position [rad] [back front]/1 -> Sum7/1
  kd/1 -> Sum9/2
  Measured Velocity [rad/s] [back front]/1 -> Sum8/2
  Desired Acceleration [rad/s^2] [back front]/1 -> Product/1
  Product/1 -> Sum1/2
  Right/Left Leg [1/0]/1 -> Friction Compensation/1(Right/Left [1/0])
  Sum2/1 -> Commanded Torque [Nm] [back front]/1
  Desired Velocity [rad/s] [back front]/1 -> Friction Compensation/2(Commanded Velocity [rad/s] [back front]), Sum8/1
  reflected inertia/1 -> Product/2
  RPM in Flight/1 -> Motor Efficiency/1(rpm)
  Motor Efficiency/1(mu) -> Divide/2
  Divide/1 -> Sum2/1
  Sum1/1 -> Divide/1
  Load Torque in Flight/1 -> Motor Efficiency/2(load_torque)

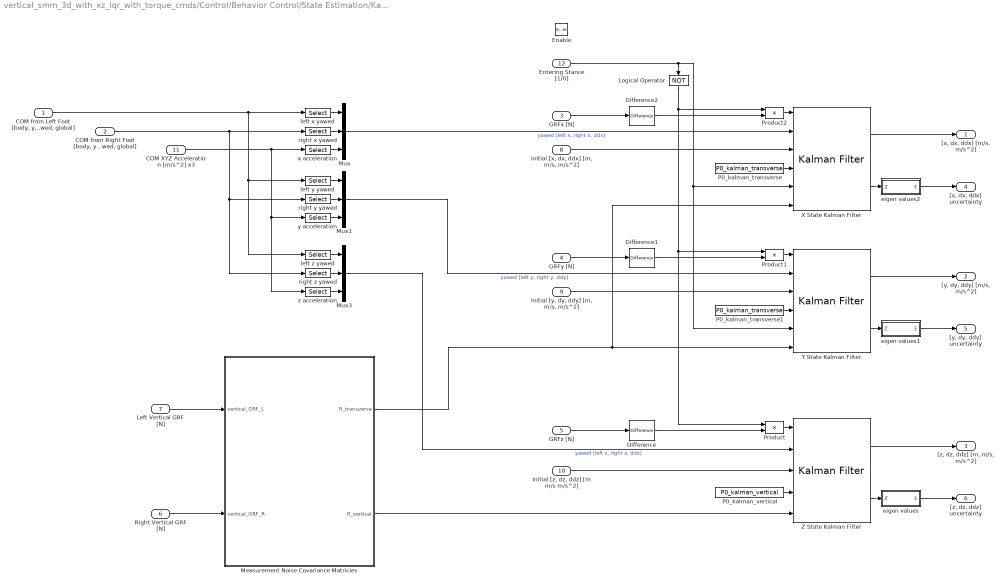
== system vertical_smm_3d_with_xz_lqr_with_torque_cmds/Control/Behavior Control/State Estimation/Kalman Filtering ==
  "COM from Left Foot [body, yawed, global]" : Inport  SampleTime=sample_time
  "COM from Right Foot [body, yawed, global]" : Inport  Port=2  SampleTime=sample_time
  GRFx [N] : Inport  Port=3  SampleTime=sample_time
  GRFy [N] : Inport  Port=4  SampleTime=sample_time
  GRFz [N] : Inport  Port=5  SampleTime=sample_time
  Right Vertical GRF [N] : Inport  Port=6  SampleTime=sample_time
  Left Vertical GRF [N] : Inport  Port=7  SampleTime=sample_time
  "Initial [x, dx, ddx] [m, m/s, m/s^2]" : Inport  Port=8  PortDimensions=3  SampleTime=sample_time
  "Initial [y, dy, ddy] [m, m/s, m/s^2]" : Inport  Port=9  PortDimensions=3  SampleTime=sample_time
  "Initial [z, dz, ddz] [m m/s m/s^2]" : Inport  Port=10  PortDimensions=3  SampleTime=sample_time
  COM XYZ Acceleration [m/s^2] x3 : Inport  Port=11  SampleTime=sample_time
  Entering Stance [1/0] : Inport  Port=12  PortDimensions=1  SampleTime=sample_time
  Enable : EnablePort  StatesWhenEnabling=reset
  Difference : simulink/Discrete/Difference  ICPrevInput=0.0  InputProcessing=Inherited  OutMin=[]  OutMax=[]  OutDataType=fixdt(1, 16)  OutScaling=2^-10  DoSatur=off
  Difference1 : simulink/Discrete/Difference  ICPrevInput=0.0  InputProcessing=Inherited  OutMin=[]  OutMax=[]  OutDataType=fixdt(1, 16)  OutScaling=2^-10  DoSatur=off
  Difference2 : simulink/Discrete/Difference  ICPrevInput=0.0  InputProcessing=Inherited  OutMin=[]  OutMax=[]  OutDataType=fixdt(1, 16)  OutScaling=2^-10  DoSatur=off
  Logical Operator : Logic  Operator=NOT  AllPortsSameDT=off  OutDataTypeStr=boolean
  Measurement Noise Covariance Matricies : MATLAB Function  TreatAsAtomicUnit=on
  Mux : Mux  Inputs=3
  Mux1 : Mux  Inputs=3
  Mux3 : Mux  Inputs=3
  P0_kalman_transverse : Constant  Value=P0_kalman_transverse
  P0_kalman_transverse1 : Constant  Value=P0_kalman_transverse
  P0_kalman_vertical : Constant  Value=P0_kalman_vertical
  Product : Product
  Product1 : Product
  Product2 : Product
  X State Kalman Filter : ctrlSharedLib/Kalman Filter  TimeDomain=Discrete-Time  UseCurrentEstimator=on  ModelSource=Individual A, B, C, D matrices  ModelSourceVariable=A_kf  A=A_kalman_transverse  B=B_kalman_transverse  C=C_kalman_transverse  D=0  NumberOfStates=2  NumberOfInputs=1  NumberOfOutputs=2  InitialEstimateSource=Input port  X0=initial_dx_estimate  P0=P0_kalman_transverse  UseK=off  UseGH=on  NumberOfProcessNoiseInputs=1  G=G_kalman_transverse  TimeInvariantG=on  H=0  TimeInvariantH=on  Q=Q_kalman_GRF_difference  TimeInvariantQ=on  R=1  TimeInvariantR=off  N=0  TimeInvariantN=on  AddInputPort=on  AddEnablePort=off  ExternalReset=Rising  OutputEstimatedY=off  OutputP=on  Ts=sample_time
  Y State Kalman Filter : ctrlSharedLib/Kalman Filter  TimeDomain=Discrete-Time  UseCurrentEstimator=on  ModelSource=Individual A, B, C, D matrices  ModelSourceVariable=A_kf  A=A_kalman_transverse  B=B_kalman_transverse  C=C_kalman_transverse  D=0  NumberOfStates=2  NumberOfInputs=1  NumberOfOutputs=2  InitialEstimateSource=Input port  X0=initial_dy_estimate  P0=P0_kalman_transverse  UseK=off  UseGH=on  NumberOfProcessNoiseInputs=1  G=G_kalman_transverse  TimeInvariantG=on  H=0  TimeInvariantH=on  Q=Q_kalman_GRF_difference  TimeInvariantQ=on  R=1  TimeInvariantR=off  N=0  TimeInvariantN=on  AddInputPort=on  AddEnablePort=off  ExternalReset=Rising  OutputEstimatedY=off  OutputP=on  Ts=sample_time
  Z State Kalman Filter : ctrlSharedLib/Kalman Filter  TimeDomain=Discrete-Time  UseCurrentEstimator=on  ModelSource=Individual A, B, C, D matrices  ModelSourceVariable=A_kf  A=A_kalman_vertical  B=B_kalman_vertical  C=C_kalman_vertical  D=0  NumberOfStates=2  NumberOfInputs=1  NumberOfOutputs=2  InitialEstimateSource=Input port  X0=[initial_z_estimate; initial_dz_estimate]  P0=P0_kalman_vertical  UseK=off  UseGH=on  NumberOfProcessNoiseInputs=1  G=G_kalman_vertical  TimeInvariantG=on  H=0  TimeInvariantH=on  Q=Q_kalman_GRF_difference  TimeInvariantQ=on  R=1  TimeInvariantR=off  N=0  TimeInvariantN=on  AddInputPort=on  AddEnablePort=off  OutputEstimatedY=off  OutputP=on  Ts=sample_time
  eigen values : MATLAB Function  TreatAsAtomicUnit=on
  eigen values1 : MATLAB Function  TreatAsAtomicUnit=on
  eigen values2 : MATLAB Function  TreatAsAtomicUnit=on
  left x yawed : Selector  InputPortWidth=9  Indices=[4]
  left y yawed : Selector  InputPortWidth=9  Indices=[5]
  left z yawed : Selector  InputPortWidth=9  Indices=[6]
  right x yawed : Selector  InputPortWidth=9  Indices=[4]
  right y yawed : Selector  InputPortWidth=9  Indices=[5]
  right z yawed : Selector  InputPortWidth=9  Indices=[6]
  x acceleration : Selector  InputPortWidth=3  Indices=[1]
  y acceleration : Selector  InputPortWidth=3  Indices=[2]
  z acceleration : Selector  InputPortWidth=3  Indices=[3]
  "[x, dx, ddx] [m/s, m/s^2]" : Outport
  "[y, dy, ddy] [m/s, m/s^2]" : Outport  Port=2
  "[z, dz, ddz] [m, m/s, m/s^2]" : Outport  Port=3
  "[x, dx, ddx] uncertainty" : Outport  Port=4
  "[y, dy, ddy] uncertainty" : Outport  Port=5
  "[z, dz, ddz] uncertainty" : Outport  Port=6
  wires:
  X State Kalman Filter/1 -> "[x, dx, ddx] [m/s, m/s^2]"/1
  eigen values1/1(E) -> "[y, dy, ddy] uncertainty"/1
  eigen values2/1(E) -> "[x, dx, ddx] uncertainty"/1
  Y State Kalman Filter/1 -> "[y, dy, ddy] [m/s, m/s^2]"/1
  y acceleration/1 -> Mux1/3
  x acceleration/1 -> Mux/3
  z acceleration/1 -> Mux3/3
  COM XYZ Acceleration [m/s^2] x3/1 -> z acceleration/1, y acceleration/1, x acceleration/1
  Z State Kalman Filter/1 -> "[z, dz, ddz] [m, m/s, m/s^2]"/1
  GRFy [N]/1 -> Difference1/1
  Mux3/1 -> Z State Kalman Filter/2  "yawed [left z, right z, ddz]"
  GRFx [N]/1 -> Difference2/1
  Measurement Noise Covariance Matricies/2(R_vertical) -> Z State Kalman Filter/5
  Measurement Noise Covariance Matricies/1(R_transverse) -> X State Kalman Filter/6, Y State Kalman Filter/6
  Mux1/1 -> Y State Kalman Filter/2  "yawed [left y, right y, ddy]"
  Mux/1 -> X State Kalman Filter/2  "yawed [left x, right x, ddx]"
  Right Vertical GRF [N]/1 -> Measurement Noise Covariance Matricies/2(vertical_GRF_R)
  Left Vertical GRF [N]/1 -> Measurement Noise Covariance Matricies/1(vertical_GRF_L)
  "COM from Left Foot [body, yawed, global]"/1 -> left z yawed/1, left y yawed/1, left x yawed/1
  left x yawed/1 -> Mux/1
  "COM from Right Foot [body, yawed, global]"/1 -> right z yawed/1, right y yawed/1, right x yawed/1
  right x yawed/1 -> Mux/2
  left y yawed/1 -> Mux1/1
  right y yawed/1 -> Mux1/2
  left z yawed/1 -> Mux3/1
  right z yawed/1 -> Mux3/2
  P0_kalman_transverse/1 -> X State Kalman Filter/4
  "Initial [x, dx, ddx] [m, m/s, m/s^2]"/1 -> X State Kalman Filter/3
  P0_kalman_transverse1/1 -> Y State Kalman Filter/4
  "Initial [y, dy, ddy] [m, m/s, m/s^2]"/1 -> Y State Kalman Filter/3
  P0_kalman_vertical/1 -> Z State Kalman Filter/4
  "Initial [z, dz, ddz] [m m/s m/s^2]"/1 -> Z State Kalman Filter/3
  X State Kalman Filter/2 -> eigen values2/1(Z)
  Y State Kalman Filter/2 -> eigen values1/1(Z)
  Z State Kalman Filter/2 -> eigen values/1(Z)
  eigen values/1(E) -> "[z, dz, ddz] uncertainty"/1
  Logical Operator/1 -> Product2/1, Product/1, Product1/1
  Difference/1 -> Product/2
  Entering Stance [1/0]/1 -> Y State Kalman Filter/5, X State Kalman Filter/5, Logical Operator/1
  Difference1/1 -> Product1/2
  Difference2/1 -> Product2/2
  Product2/1 -> X State Kalman Filter/1
  Product1/1 -> Y State Kalman Filter/1
  Product/1 -> Z State Kalman Filter/1
  GRFz [N]/1 -> Difference/1

== system vertical_smm_3d_with_xz_lqr_with_torque_cmds/Control/Behavior Control/Primary and Lateral Behavior/Circular Buffer/Enabled on Touchdown ==
  In : Inport
  Enable : EnablePort
  Out : Outport
  wires:
  In/1 -> Out/1

== system vertical_smm_3d_with_xz_lqr_with_torque_cmds/Control/Behavior Control/Primary and Lateral Behavior/Flight/Back//Front Motor PD ==
  Desired Position [rad] [back front] : Inport
  Desired Velocity [rad/s] [back front] : Inport  Port=2
  Desired Acceleration [rad/s^2] [back front] : Inport  Port=3
  Measured Position [rad] [back front] : Inport  Port=4
  Measured Velocity [rad/s] [back front] : Inport  Port=5
  Right/Left Leg [1/0] : Inport  Port=6
  Divide : Product  Inputs=*/
  Friction Compensation : Subsystem
  Load Torque in Flight : Constant  Value=30
  Motor Efficiency : MATLAB Function  TreatAsAtomicUnit=on
  Product : Product
  RadPerSecToRotorRpm : Gain  Gain=60*LEG_MTR_GEAR_RATIO/(2*pi)
  Sum1 : Sum  Inputs=|++
  Sum2 : Sum  Inputs=|++
  Sum7 : Sum  Inputs=|+-
  Sum8 : Sum  Inputs=|+-
  Sum9 : Sum
  kd : Gain  Gain=kd_motor
  kp : Gain  Gain=kp_motor
  reflected inertia : Constant  Value=j_motor
  Commanded Torque [Nm] [back front] : Outport
  wires:
  kp/1 -> Sum9/1
  Sum7/1 -> kp/1
  Measured Position [rad] [back front]/1 -> Sum7/2
  Sum9/1 -> Sum1/1
  Sum8/1 -> kd/1
  Desired Position [rad] [back front]/1 -> Sum7/1
  kd/1 -> Sum9/2
  Measured Velocity [rad/s] [back front]/1 -> Sum8/2
  Desired Acceleration [rad/s^2] [back front]/1 -> Product/1
  Product/1 -> Sum1/2
  Right/Left Leg [1/0]/1 -> Friction Compensation/1(Right/Left [1/0])
  Sum2/1 -> Commanded Torque [Nm] [back front]/1
  Desired Velocity [rad/s] [back front]/1 -> RadPerSecToRotorRpm/1, Friction Compensation/2(Commanded Velocity [rad/s] [back front]), Sum8/1
  reflected inertia/1 -> Product/2
  Friction Compensation/1(Friction Compensation [Nm]) -> Sum2/2
  RadPerSecToRotorRpm/1 -> Motor Efficiency/1(rpm)
  Motor Efficiency/1(mu) -> Divide/2
  Divide/1 -> Sum2/1
  Sum1/1 -> Divide/1
  Load Torque in Flight/1 -> Motor Efficiency/2(load_torque)

== system vertical_smm_3d_with_xz_lqr_with_torque_cmds/Control/Behavior Control/Primary and Lateral Behavior/Flight/Hold Values on Takeoff ==
  in : Inport
  Trigger : TriggerPort  ShowOutputPort=on  PortDimensions=1
  Subsystem : Subsystem
  out : Outport
  wires:
  Trigger/1 -> Subsystem/Enable
  Subsystem/1(out) -> out/1
  in/1 -> Subsystem/1(in)

== system vertical_smm_3d_with_xz_lqr_with_torque_cmds/Control/Behavior Control/Primary and Lateral Behavior/Stance/Chirp Frequency ==
  Time Since Stance : Inport
  Chirp Freq Factor Saturation : Saturate  UpperLimit=4  LowerLimit=0
      settings: AttributesFormatString=Top: %<UpperLimit>\nBottom: %<LowerLimit>
  Compare To Constant1 : simulink/Logic and Bit Operations/Compare To Constant  relop=~=  const=4  OutDataTypeStr=boolean
  Constant1 : Constant
  Constant5 : Constant  Value=0.075
  Product{1..4} (4 alike) : Product
  Sum : Sum  Inputs=++|
  standing_bounce_frequency : Constant  Value=standing_bounce_frequency
  w : Outport
  dw/dt : Outport  Port=2
  wires:
  Constant1/1 -> Sum/1
  Product4/1 -> Sum/2
  Sum/1 -> Chirp Freq Factor Saturation/1
  Time Since Stance/1 -> Product4/1
  Constant5/1 -> Product4/2, Product2/2
  Product2/1 -> Product1/2
  Compare To Constant1/1 -> Product1/1
  Product1/1 -> dw/dt/1
  Product3/1 -> w/1
  Chirp Freq Factor Saturation/1 -> Compare To Constant1/1, Product3/2
  standing_bounce_frequency/1 -> Product3/1, Product2/1

== system vertical_smm_3d_with_xz_lqr_with_torque_cmds/Control/Behavior Control/Primary and Lateral Behavior/Stance/Compute Forces ==
  XYZ Acceleration : Inport
  Constant5 : Constant  Value=g
  Demux : Demux  Outputs=3
  Gain4 : Gain  Gain=m_total_real
  Mux : Mux  Inputs=3
  Sum8 : Sum  Inputs=|++
  XYZ Force : Outport
  wires:
  Demux/1 -> Mux/1
  Demux/2 -> Mux/2
  Demux/3 -> Sum8/1
  Sum8/1 -> Mux/3
  Mux/1 -> Gain4/1
  Gain4/1 -> XYZ Force/1
  XYZ Acceleration/1 -> Demux/1
  Constant5/1 -> Sum8/2
